simulink library "HexapodLocomotion_Library"  (R2023a)
settings: Solver=VariableStepAuto  StartTime=0.0  StopTime=10.0  RelTol=1e-3
values from neighbouring files (symbols this model uses):
  AEP = 0.03    [simulation_setup.m]
  max_torque_alpha = globalTorque    (= 0.94)    [InitialisationScript.m]    (also in simulation_setup.m)
  max_torque_beta = globalTorque    (= 0.94)    [InitialisationScript.m]    (also in simulation_setup.m)
  max_torque_gamma = globalTorque    (= 0.94)    [InitialisationScript.m]    (also in simulation_setup.m)
  N = 16    [rl_setup.m]
  PEP = -0.03    [simulation_setup.m]
  pid_D = 1    [InitialisationScript.m]    (also in simulation_setup.m)
  pid_filter_N = 100    [InitialisationScript.m]    (also in simulation_setup.m = 1000)
  pid_I = 0.2    [InitialisationScript.m]    (also in simulation_setup.m = 0.1)
  pid_P = 3    [InitialisationScript.m]    (also in simulation_setup.m = 600)
  step_height = 0.06    [InitialisationScript.m]    (also in simulation_setup.m)
  step_length = 0.04    [InitialisationScript.m]    (also in simulation_setup.m)
undefined symbols (not defined in the file or in its folder): X, Y, Z
libraries: sm_lib x31, nesl_utility x13, $bdroot x5, slpidlib x3
(part 1 of 2)
settings Model: Creator=basti  LastModifiedBy=basti

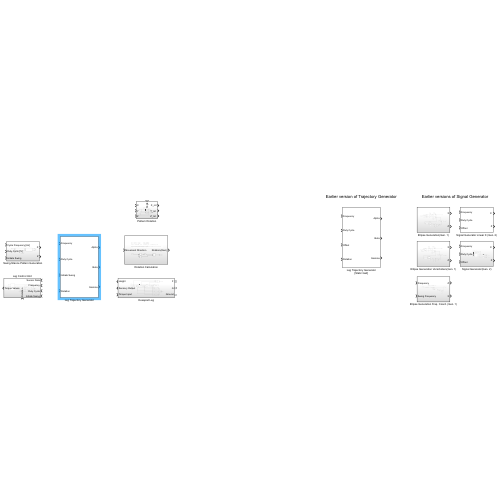
[thumbnail: Simulink's stored preview of the top-level diagram]
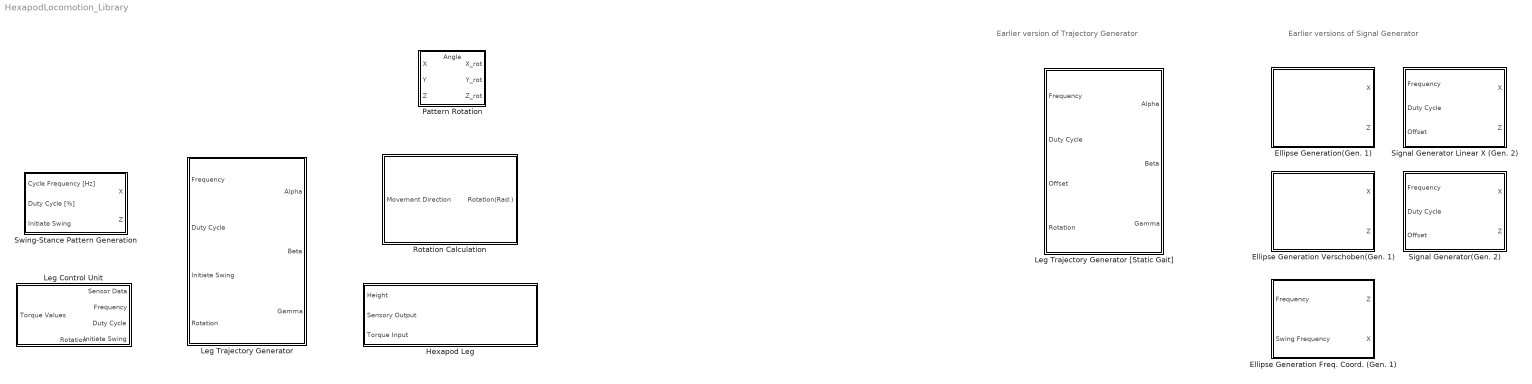
== system HexapodLocomotion_Library ==
  note: Earlier versions of Signal Generator
  note: Earlier version of Trajectory Generator
  Ellipse Generation Freq. Coord. (Gen. 1) : Subsystem
  Ellipse Generation Verschoben(Gen. 1) : Subsystem
  Ellipse Generation(Gen. 1) : Subsystem
  Hexapod Leg : Subsystem
      settings: PortSchema="{\"entries\":[{\"content\":{\"sides\":[{\"content\":{\"connectorIds\":[\"LConn1\",\"LConn2\",\"LConn3\"]},\"type\":\"ConnectorPlacement.EquallySpacedRectSide\",\"uuid\":\"f49879d6-ba76-4ec0-9cde-e27e7d64cb43\"},{\"content\":{\"connectorIds\":[\"In1\",\"Out1\",\"Out2\"],\"side\":\"RIGHT\"},\"type\":\"ConnectorPlacement.EquallySpacedRectSide\",\"uuid\":\"65b15dde-e5d7-47cb-8ac1-e9e029e05721\"},{\"content\":{\"side\":\"TOP\"},\"type\":\"ConnectorPlacement.EquallySpacedRectSide\",\"uuid\":\"11559e5b-a1be-4233-aeb2-21e170c4e963\"}]},\"type\":\"ConnectorPlacement.EquallySpacedConnector\",\"uuid\":\"c4377ad5-9946-4ac5-9145-d9e25f76b3b4\"}],\"packageUris\":[\"http://schema.mathworks.com/mf0/Connector/R2020b\"],\"version\":\"1.0\"}"
  Leg Control Unit : Subsystem
      settings: PortSchema="{\"entries\":[{\"content\":{\"sides\":[{\"content\":{\"connectorIds\":[\"In1\",\"In2\",\"In3\",\"In4\"]},\"type\":\"ConnectorPlacement.EquallySpacedRectSide\",\"uuid\":\"61807659-790a-4fcc-8eea-bb1747959d2c\"},{\"content\":{\"connectorIds\":[\"Out1\"],\"side\":\"RIGHT\"},\"type\":\"ConnectorPlacement.EquallySpacedRectSide\",\"uuid\":\"beab48f8-df50-4720-a4fe-1084d91255e1\"},{\"content\":{\"side\":\"TOP\"},\"type\":\"ConnectorPlacement.EquallySpacedRectSide\",\"uuid\":\"df2f0e11-b286-4413-8948-937711258f59\"},{\"content\":{\"connectorIds\":[\"In5\"],\"side\":\"BOTTOM\"},\"type\":\"ConnectorPlacement.EquallySpacedRectSide\",\"uuid\":\"177fd513-fdd6-4ae0-8805-86acc5cb073f\"}]},\"type\":\"ConnectorPlacement.EquallySpacedConnector\",\"uuid\":\"735c34ff-c8fb-4d96-b4d8-f985913f524f\"}],\"packageUris\":[\"http://schema.mathworks.com/mf0/Connector/R2020b\"],\"version\":\"1.0\"}"
  Leg Trajectory Generator : Subsystem  mask{step_height=0, step_length=0, x_offset=0, y_offset=0, z_offset=0, angle_offsets=0}
      mask prompts: step_height "Step Length"; step_length "Step Height"; x_offset "x-Offset"; y_offset "y-Offset"; z_offset "z-Offset"; angle_offsets "Angle Offsets"
  Leg Trajectory Generator [Static Gait] : Subsystem  mask{step_height=0, step_length=0, x_offset=0, y_offset=0, z_offset=0, angle_offsets=0}
      mask prompts: step_height "Step Length"; step_length "Step Height"; x_offset "x-Offset"; y_offset "y-Offset"; z_offset "z-Offset"; angle_offsets "Angle Offsets"
  Pattern Rotation : Subsystem
      settings: PortSchema="{\"entries\":[{\"content\":{\"sides\":[{\"content\":{\"connectorIds\":[\"In1\",\"In2\",\"In3\"]},\"type\":\"ConnectorPlacement.EquallySpacedRectSide\",\"uuid\":\"84b9b2e7-3aec-4c44-82b0-943baf46ecad\"},{\"content\":{\"connectorIds\":[\"Out1\",\"Out2\",\"Out3\"],\"side\":\"RIGHT\"},\"type\":\"ConnectorPlacement.EquallySpacedRectSide\",\"uuid\":\"b6460351-c898-40bb-b6f7-4663874c85b4\"},{\"content\":{\"connectorIds\":[\"In4\"],\"side\":\"TOP\"},\"type\":\"ConnectorPlacement.EquallySpacedRectSide\",\"uuid\":\"52dfc046-6500-4cf8-9639-535088e7a0e1\"}]},\"type\":\"ConnectorPlacement.EquallySpacedConnector\",\"uuid\":\"f9a3b501-bdbb-45c4-9129-59c2d41cd802\"}],\"packageUris\":[\"http://schema.mathworks.com/mf0/Connector/R2020b\"],\"version\":\"1.0\"}"
  Rotation Calculation : Subsystem
  Signal Generator Linear X (Gen. 2) : Subsystem  mask{x_amplitude=0, z_amplitude=0}
      mask prompts: x_amplitude "x-Amplitude"; z_amplitude "z-Amplitude"
  Signal Generator(Gen. 2) : Subsystem
  Swing-Stance Pattern Generation : Subsystem

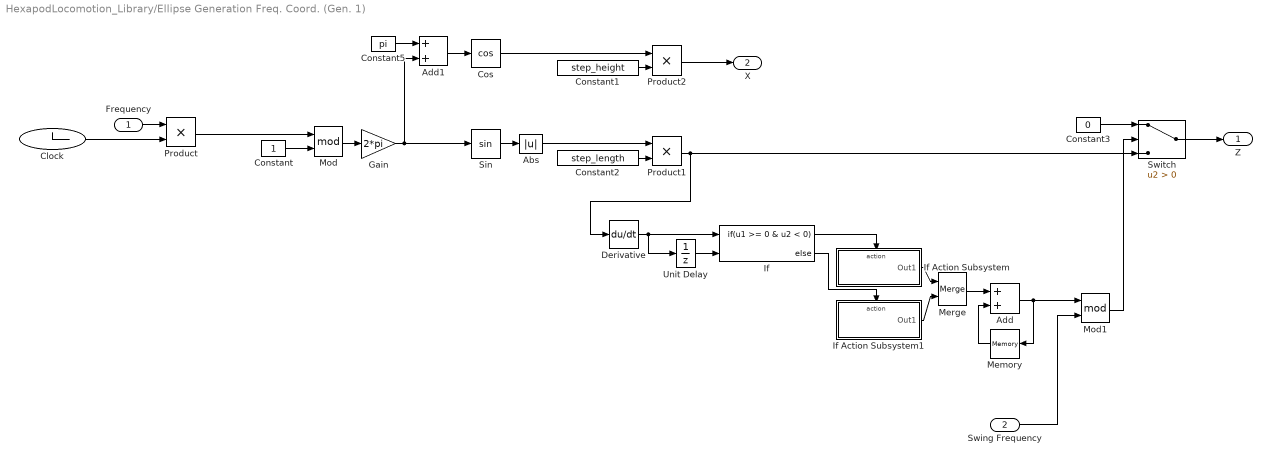
== system HexapodLocomotion_Library/Ellipse Generation Freq. Coord. (Gen. 1) ==
  Frequency : Inport
  Swing Frequency : Inport  Port=2
  Abs : Abs  SaturateOnIntegerOverflow=off
  Add : Sum
  Add1 : Sum
  Clock : Clock
  Constant : Constant
  Constant1 : Constant  Value=step_height
  Constant2 : Constant  Value=step_length
  Constant3 : Constant  Value=0
  Constant5 : Constant  Value=pi
  Cos : Trigonometry  Operator=cos
  Derivative : Derivative
  Gain : Gain  Gain=2*pi
  If : If  NumInputs=2  IfExpression=u1 >= 0 & u2 < 0
  If Action Subsystem : Subsystem  TreatAsAtomicUnit=on
  If Action Subsystem1 : Subsystem  TreatAsAtomicUnit=on
  Memory : Memory
  Merge : Merge
  Mod : Math  Operator=mod
  Mod1 : Math  Operator=mod
  Product : Product
  Product1 : Product
  Product2 : Product
  Sin : Trigonometry
  Switch : Switch  Criteria=u2 > Threshold  SaturateOnIntegerOverflow=off  InputSameDT=off
  Unit Delay : UnitDelay  SampleTime=-1  HasFrameUpgradeWarning=on
  Z : Outport
  X : Outport  Port=2
  wires:
  Clock/1 -> Product/2
  Frequency/1 -> Product/1
  Product/1 -> Mod/1
  Constant/1 -> Mod/2
  Mod/1 -> Gain/1
  Sin/1 -> Abs/1
  Constant2/1 -> Product1/2
  Cos/1 -> Product2/1
  Constant1/1 -> Product2/2
  Product1/1 -> Switch/3, Derivative/1
  Constant3/1 -> Switch/1
  Abs/1 -> Product1/1
  Derivative/1 -> Unit Delay/1, If/1
  Unit Delay/1 -> If/2
  If/2 -> If Action Subsystem1/Action
  If/1 -> If Action Subsystem/Action
  If Action Subsystem/1(Out1) -> Merge/1
  If Action Subsystem1/1(Out1) -> Merge/2
  Switch/1 -> Z/1
  Product2/1 -> X/1
  Merge/1 -> Add/1
  Memory/1 -> Add/2
  Add/1 -> Mod1/1, Memory/1
  Swing Frequency/1 -> Mod1/2
  Mod1/1 -> Switch/2
  Add1/1 -> Cos/1
  Constant5/1 -> Add1/1
  Gain/1 -> Add1/2, Sin/1

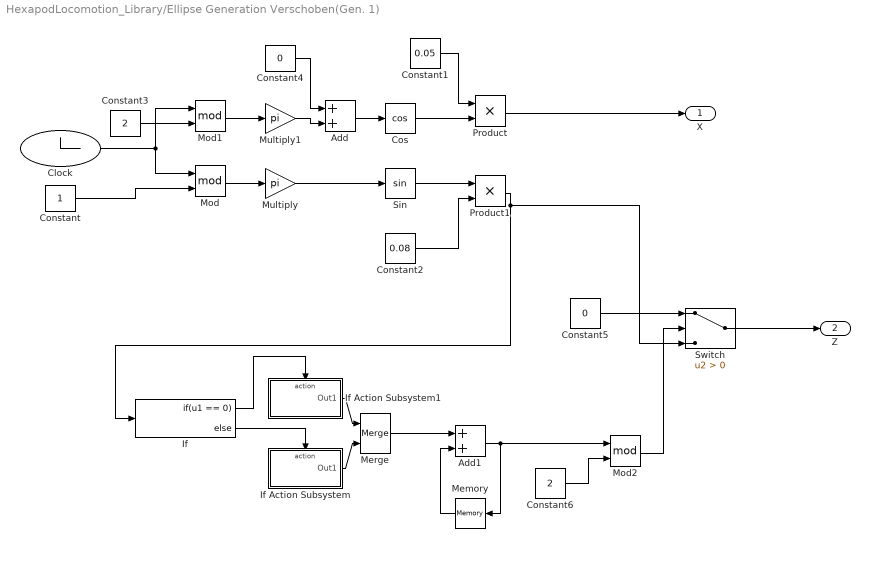
== system HexapodLocomotion_Library/Ellipse Generation Verschoben(Gen. 1) ==
  Add : Sum
  Add1 : Sum
  Clock : Clock
  Constant : Constant
  Constant1 : Constant  Value=0.05
  Constant2 : Constant  Value=0.08
  Constant3 : Constant  Value=2
  Constant4 : Constant  Value=0
  Constant5 : Constant  Value=0
  Constant6 : Constant  Value=2
  Cos : Trigonometry  Operator=cos
  If : If  IfExpression=u1 == 0
  If Action Subsystem : Subsystem  TreatAsAtomicUnit=on
  If Action Subsystem1 : Subsystem  TreatAsAtomicUnit=on
  Memory : Memory
  Merge : Merge
  Mod : Math  Operator=mod
  Mod1 : Math  Operator=mod
  Mod2 : Math  Operator=mod
  Multiply : Gain  Gain=pi
  Multiply1 : Gain  Gain=pi
  Product : Product
  Product1 : Product
  Sin : Trigonometry
  Switch : Switch  Criteria=u2 > Threshold  SaturateOnIntegerOverflow=off  InputSameDT=off
  X : Outport
  Z : Outport  Port=2
  wires:
  Clock/1 -> Mod1/1, Mod/1
  Constant/1 -> Mod/2
  Mod/1 -> Multiply/1
  Multiply/1 -> Sin/1
  Sin/1 -> Product1/1
  Cos/1 -> Product/2
  Constant1/1 -> Product/1
  Constant2/1 -> Product1/2
  Product1/1 -> Switch/3, If/1
  Product/1 -> X/1
  Mod1/1 -> Multiply1/1
  Constant3/1 -> Mod1/2
  Add/1 -> Cos/1
  Multiply1/1 -> Add/2
  Constant4/1 -> Add/1
  Add1/1 -> Mod2/1, Memory/1
  Memory/1 -> Add1/2
  If/2 -> If Action Subsystem/Action
  If/1 -> If Action Subsystem1/Action
  If Action Subsystem/1(Out1) -> Merge/2
  If Action Subsystem1/1(Out1) -> Merge/1
  Merge/1 -> Add1/1
  Switch/1 -> Z/1
  Constant5/1 -> Switch/1
  Constant6/1 -> Mod2/2
  Mod2/1 -> Switch/2

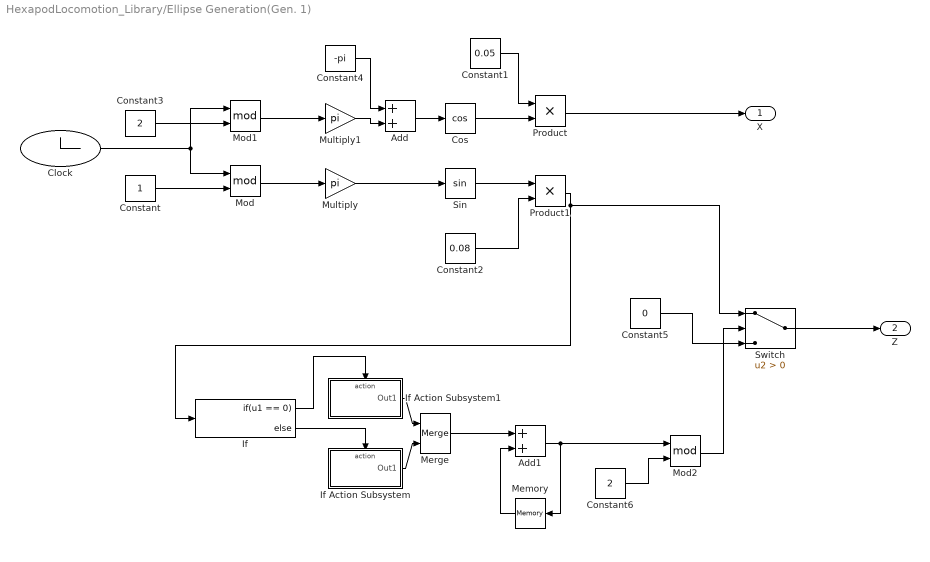
== system HexapodLocomotion_Library/Ellipse Generation(Gen. 1) ==
  Add : Sum
  Add1 : Sum
  Clock : Clock
  Constant : Constant
  Constant1 : Constant  Value=0.05
  Constant2 : Constant  Value=0.08
  Constant3 : Constant  Value=2
  Constant4 : Constant  Value=-pi
  Constant5 : Constant  Value=0
  Constant6 : Constant  Value=2
  Cos : Trigonometry  Operator=cos
  If : If  IfExpression=u1 == 0
  If Action Subsystem : Subsystem  TreatAsAtomicUnit=on
  If Action Subsystem1 : Subsystem  TreatAsAtomicUnit=on
  Memory : Memory
  Merge : Merge
  Mod : Math  Operator=mod
  Mod1 : Math  Operator=mod
  Mod2 : Math  Operator=mod
  Multiply : Gain  Gain=pi
  Multiply1 : Gain  Gain=pi
  Product : Product
  Product1 : Product
  Sin : Trigonometry
  Switch : Switch  Criteria=u2 > Threshold  SaturateOnIntegerOverflow=off  InputSameDT=off
  X : Outport
  Z : Outport  Port=2
  wires:
  Clock/1 -> Mod1/1, Mod/1
  Constant/1 -> Mod/2
  Mod/1 -> Multiply/1
  Multiply/1 -> Sin/1
  Sin/1 -> Product1/1
  Cos/1 -> Product/2
  Constant1/1 -> Product/1
  Constant2/1 -> Product1/2
  Product1/1 -> Switch/1, If/1
  Product/1 -> X/1
  Mod1/1 -> Multiply1/1
  Constant3/1 -> Mod1/2
  Add/1 -> Cos/1
  Multiply1/1 -> Add/2
  Constant4/1 -> Add/1
  Add1/1 -> Mod2/1, Memory/1
  Memory/1 -> Add1/2
  If/2 -> If Action Subsystem/Action
  If/1 -> If Action Subsystem1/Action
  If Action Subsystem/1(Out1) -> Merge/2
  If Action Subsystem1/1(Out1) -> Merge/1
  Merge/1 -> Add1/1
  Switch/1 -> Z/1
  Constant5/1 -> Switch/3
  Constant6/1 -> Mod2/2
  Mod2/1 -> Switch/2

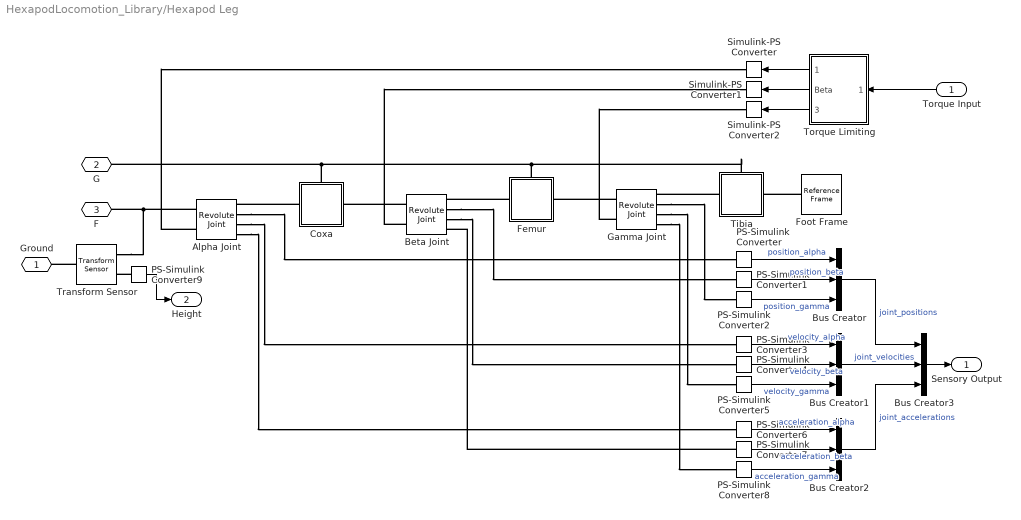
== system HexapodLocomotion_Library/Hexapod Leg ==
  Torque Input : Inport
  Alpha Joint : sm_lib/Joints/Revolute Joint  JointMode=Normal  SenseConstraintForce=off  SenseConstraintForceX=off  SenseConstraintForceY=off  SenseConstraintForceZ=off  SenseConstraintTorque=off  SenseConstraintTorqueX=off  SenseConstraintTorqueY=off  SenseConstraintTorqueZ=off  SenseTotalForce=off  SenseTotalForceX=off  SenseTotalForceY=off  SenseTotalForceZ=off  SenseTotalTorque=off  SenseTotalTorqueX=off  SenseTotalTorqueY=off  SenseTotalTorqueZ=off  CompositeWrenchDir=FollowerOnBase  CompositeWrenchFrame=BaseFrame  EquilibriumPosition=0  EquilibriumPositionUnits=deg  SpringStiffness=0  SpringStiffnessUnits=N*m/deg  DampingCoefficient=joint_damping_coefficient  DampingCoefficientUnits=kg*m^2/(rad*s)  TorqueActuationMode=InputTorque  MotionActuationMode=ComputedMotion  SensePosition=on  SenseVelocity=on  SenseAcceleration=on  SenseTorqueForce=off  SenseLowerLimitTorqueForce=off  SenseUpperLimitTorqueForce=off  LowerLimitSpecify=on  LowerLimitBound=-0.9599310885968813  LowerLimitBoundUnits=rad  LowerLimitStiffness=1e4  LowerLimitStiffnessUnits=N*m/deg  LowerLimitDamping=10  LowerLimitDampingUnits=N*m/(deg/s)  LowerLimitTransitionRegionWidth=global_transition_region  LowerLimitTransitionRegionWidthUnits=deg  UpperLimitSpecify=on  UpperLimitBound=0.9599310885968813  UpperLimitBoundUnits=rad  UpperLimitStiffness=1e4  UpperLimitStiffnessUnits=N*m/deg  UpperLimitDamping=10  UpperLimitDampingUnits=N*m/(deg/s)  UpperLimitTransitionRegionWidth=global_transition_region  UpperLimitTransitionRegionWidthUnits=deg  PositionTargetSpecify=on  PositionTargetPriority=High  PositionTargetValue=0  PositionTargetValueUnits=rad  VelocityTargetSpecify=off  VelocityTargetPriority=High  VelocityTargetValue=0  VelocityTargetValueUnits=deg/s
  Beta Joint : sm_lib/Joints/Revolute Joint  JointMode=Normal  SenseConstraintForce=off  SenseConstraintForceX=off  SenseConstraintForceY=off  SenseConstraintForceZ=off  SenseConstraintTorque=off  SenseConstraintTorqueX=off  SenseConstraintTorqueY=off  SenseConstraintTorqueZ=off  SenseTotalForce=off  SenseTotalForceX=off  SenseTotalForceY=off  SenseTotalForceZ=off  SenseTotalTorque=off  SenseTotalTorqueX=off  SenseTotalTorqueY=off  SenseTotalTorqueZ=off  CompositeWrenchDir=FollowerOnBase  CompositeWrenchFrame=BaseFrame  EquilibriumPosition=0  EquilibriumPositionUnits=deg  SpringStiffness=0  SpringStiffnessUnits=N*m/deg  DampingCoefficient=joint_damping_coefficient  DampingCoefficientUnits=kg*m^2/(rad*s)  TorqueActuationMode=InputTorque  MotionActuationMode=ComputedMotion  SensePosition=on  SenseVelocity=on  SenseAcceleration=on  SenseTorqueForce=off  SenseLowerLimitTorqueForce=off  SenseUpperLimitTorqueForce=off  LowerLimitSpecify=on  LowerLimitBound=-1.710422666954443  LowerLimitBoundUnits=rad  LowerLimitStiffness=1e4  LowerLimitStiffnessUnits=N*m/deg  LowerLimitDamping=10  LowerLimitDampingUnits=N*m/(deg/s)  LowerLimitTransitionRegionWidth=global_transition_region  LowerLimitTransitionRegionWidthUnits=deg  UpperLimitSpecify=on  UpperLimitBound=1.570796326794897  UpperLimitBoundUnits=rad  UpperLimitStiffness=1e4  UpperLimitStiffnessUnits=N*m/deg  UpperLimitDamping=10  UpperLimitDampingUnits=N*m/(deg/s)  UpperLimitTransitionRegionWidth=global_transition_region  UpperLimitTransitionRegionWidthUnits=deg  PositionTargetSpecify=on  PositionTargetPriority=High  PositionTargetValue=0  PositionTargetValueUnits=rad  VelocityTargetSpecify=off  VelocityTargetPriority=High  VelocityTargetValue=0  VelocityTargetValueUnits=deg/s
  Bus Creator{,1..3} (4 alike) : BusCreator  Inputs=3
  Coxa : Subsystem
      settings: PortSchema="{\"entries\":[{\"content\":{\"sides\":[{\"content\":{\"connectorIds\":[\"LConn1\"]},\"type\":\"ConnectorPlacement.EquallySpacedRectSide\",\"uuid\":\"688cd827-d904-4215-b5db-99d415378c46\"},{\"content\":{\"connectorIds\":[\"RConn1\"],\"side\":\"RIGHT\"},\"type\":\"ConnectorPlacement.EquallySpacedRectSide\",\"uuid\":\"69dd1601-faac-4bb0-843f-c649d8ea5326\"},{\"content\":{\"connectorIds\":[\"LConn2\"],\"side\":\"TOP\"},\"type\":\"ConnectorPlacement.EquallySpacedRectSide\",\"uuid\":\"f0d3334d-4e2f-4a21-b3dd-fad9d1fa7157\"}]},\"type\":\"ConnectorPlacement.EquallySpacedConnector\",\"uuid\":\"68f70a25-3d71-4639-b68a-a87509eaa3ad\"}],\"packageUris\":[\"http://schema.mathworks.com/mf0/Connector/R2020b\"],\"version\":\"1.0\"}"
  Femur : Subsystem
      settings: PortSchema="{\"entries\":[{\"content\":{\"sides\":[{\"content\":{\"connectorIds\":[\"LConn1\"]},\"type\":\"ConnectorPlacement.EquallySpacedRectSide\",\"uuid\":\"688cd827-d904-4215-b5db-99d415378c46\"},{\"content\":{\"connectorIds\":[\"RConn1\"],\"side\":\"RIGHT\"},\"type\":\"ConnectorPlacement.EquallySpacedRectSide\",\"uuid\":\"69dd1601-faac-4bb0-843f-c649d8ea5326\"},{\"content\":{\"connectorIds\":[\"LConn2\"],\"side\":\"TOP\"},\"type\":\"ConnectorPlacement.EquallySpacedRectSide\",\"uuid\":\"f0d3334d-4e2f-4a21-b3dd-fad9d1fa7157\"}]},\"type\":\"ConnectorPlacement.EquallySpacedConnector\",\"uuid\":\"68f70a25-3d71-4639-b68a-a87509eaa3ad\"}],\"packageUris\":[\"http://schema.mathworks.com/mf0/Connector/R2020b\"],\"version\":\"1.0\"}"
  Foot Frame : sm_lib/Frames and Transforms/Reference Frame
  Gamma Joint : sm_lib/Joints/Revolute Joint  JointMode=Normal  SenseConstraintForce=off  SenseConstraintForceX=off  SenseConstraintForceY=off  SenseConstraintForceZ=off  SenseConstraintTorque=off  SenseConstraintTorqueX=off  SenseConstraintTorqueY=off  SenseConstraintTorqueZ=off  SenseTotalForce=off  SenseTotalForceX=off  SenseTotalForceY=off  SenseTotalForceZ=off  SenseTotalTorque=off  SenseTotalTorqueX=off  SenseTotalTorqueY=off  SenseTotalTorqueZ=off  CompositeWrenchDir=FollowerOnBase  CompositeWrenchFrame=BaseFrame  EquilibriumPosition=0  EquilibriumPositionUnits=deg  SpringStiffness=0  SpringStiffnessUnits=N*m/deg  DampingCoefficient=joint_damping_coefficient  DampingCoefficientUnits=kg*m^2/(rad*s)  TorqueActuationMode=InputTorque  MotionActuationMode=ComputedMotion  SensePosition=on  SenseVelocity=on  SenseAcceleration=on  SenseTorqueForce=off  SenseLowerLimitTorqueForce=off  SenseUpperLimitTorqueForce=off  LowerLimitSpecify=on  LowerLimitBound=-0.7853981633974483  LowerLimitBoundUnits=rad  LowerLimitStiffness=1e4  LowerLimitStiffnessUnits=N*m/deg  LowerLimitDamping=10  LowerLimitDampingUnits=N*m/(deg/s)  LowerLimitTransitionRegionWidth=global_transition_region  LowerLimitTransitionRegionWidthUnits=deg  UpperLimitSpecify=on  UpperLimitBound=2.181661564992912  UpperLimitBoundUnits=rad  UpperLimitStiffness=1e4  UpperLimitStiffnessUnits=N*m/deg  UpperLimitDamping=10  UpperLimitDampingUnits=N*m/(deg/s)  UpperLimitTransitionRegionWidth=global_transition_region  UpperLimitTransitionRegionWidthUnits=deg  PositionTargetSpecify=on  PositionTargetPriority=High  PositionTargetValue=0  PositionTargetValueUnits=rad  VelocityTargetSpecify=off  VelocityTargetPriority=High  VelocityTargetValue=0  VelocityTargetValueUnits=deg/s
  PS-Simulink Converter{,1..9} (10 alike) : nesl_utility/PS-Simulink Converter  PhysicalDomain=network_engine_domain  SubClassName=ps_output  LeftPortType=input  RightPortType=output  PseudoPeriodic=off  Frequencies=[]  VectorFormat=inherit  Unit=inherit  AffineConversion=off
  Simulink-PS Converter : nesl_utility/Simulink-PS Converter  PhysicalDomain=network_engine_domain  SubClassName=ps_input  LeftPortType=input  RightPortType=output  PseudoPeriodic=off  Frequencies=[]  NoiseDistribution=none  NoiseParameters=[]  Unit=1  AffineConversion=off  FilteringAndDerivatives=provide  SimscapeFilterOrder=1  InputFilterTimeConstant=0.001  UdotUserProvided=0
  Simulink-PS Converter1 : nesl_utility/Simulink-PS Converter  PhysicalDomain=network_engine_domain  SubClassName=ps_input  LeftPortType=input  RightPortType=output  PseudoPeriodic=off  Frequencies=[]  NoiseDistribution=none  NoiseParameters=[]  Unit=1  AffineConversion=off  FilteringAndDerivatives=provide  SimscapeFilterOrder=1  InputFilterTimeConstant=0.001  UdotUserProvided=0
  Simulink-PS Converter2 : nesl_utility/Simulink-PS Converter  PhysicalDomain=network_engine_domain  SubClassName=ps_input  LeftPortType=input  RightPortType=output  PseudoPeriodic=off  Frequencies=[]  NoiseDistribution=none  NoiseParameters=[]  Unit=1  AffineConversion=off  FilteringAndDerivatives=provide  SimscapeFilterOrder=1  InputFilterTimeConstant=0.001  UdotUserProvided=0
  Tibia : Subsystem
      settings: PortSchema="{\"entries\":[{\"content\":{\"sides\":[{\"content\":{\"connectorIds\":[\"LConn1\"]},\"type\":\"ConnectorPlacement.EquallySpacedRectSide\",\"uuid\":\"99a4fa88-2354-49bd-896b-e43e2625a35e\"},{\"content\":{\"connectorIds\":[\"RConn1\"],\"side\":\"RIGHT\"},\"type\":\"ConnectorPlacement.EquallySpacedRectSide\",\"uuid\":\"27b73151-d7dc-445f-a6d8-c3ae4140e18d\"},{\"content\":{\"connectorIds\":[\"LConn2\"],\"side\":\"TOP\"},\"type\":\"ConnectorPlacement.EquallySpacedRectSide\",\"uuid\":\"5ff52d7d-b215-4137-a6c5-45615f920964\"}]},\"type\":\"ConnectorPlacement.EquallySpacedConnector\",\"uuid\":\"86768a5d-0bed-4b52-bc94-3bd267854b00\"}],\"packageUris\":[\"http://schema.mathworks.com/mf0/Connector/R2020b\"],\"version\":\"1.0\"}"
  Torque Limiting : Subsystem
  Transform Sensor : sm_lib/Frames and Transforms/Transform Sensor  MeasurementFrame=World  RotationSequence=XYX  SenseAngle=off  SenseAxis=off  SenseQ=off  SenseR=off  SenseRotationSequence=off  SenseOmegaX=off  SenseOmegaY=off  SenseOmegaZ=off  SenseQDot=off  SenseRDot=off  SenseRotationSequenceDot=off  SenseAlphaX=off  SenseAlphaY=off  SenseAlphaZ=off  SenseQDDot=off  SenseRDDot=off  SenseX=off  SenseY=off  SenseZ=on  SenseRad=off  SenseAzim=off  SenseDist=off  SenseInc=off  SenseXDot=off  SenseYDot=off  SenseZDot=off  SenseRadDot=off  SenseAzimDot=off  SenseDistDot=off  SenseIncDot=off  SenseXDDot=off  SenseYDDot=off  SenseZDDot=off  SenseRadDDot=off  SenseAzimDDot=off  SenseDistDDot=off  SenseIncDDot=off
  Ground : PMIOPort  Side=Left
  G : PMIOPort  Port=2  Side=Left
  F : PMIOPort  Port=3  Side=Left
  Sensory Output : Outport
  Height : Outport  Port=2
  wires:
  Torque Input/1 -> Torque Limiting/1(Input)
  Torque Limiting/1(Alpha) -> Simulink-PS Converter/1
  Torque Limiting/2(Beta) -> Simulink-PS Converter1/1
  Torque Limiting/3(Gamma) -> Simulink-PS Converter2/1
  PS-Simulink Converter/1 -> Bus Creator/1  "position_alpha"
  PS-Simulink Converter1/1 -> Bus Creator/2  "position_beta"
  PS-Simulink Converter2/1 -> Bus Creator/3  "position_gamma"
  PS-Simulink Converter3/1 -> Bus Creator1/1  "velocity_alpha"
  PS-Simulink Converter4/1 -> Bus Creator1/2  "velocity_beta"
  PS-Simulink Converter5/1 -> Bus Creator1/3  "velocity_gamma"
  PS-Simulink Converter6/1 -> Bus Creator2/1  "acceleration_alpha"
  PS-Simulink Converter7/1 -> Bus Creator2/2  "acceleration_beta"
  PS-Simulink Converter8/1 -> Bus Creator2/3  "acceleration_gamma"
  Bus Creator1/1 -> Bus Creator3/2  "joint_velocities"
  Bus Creator3/1 -> Sensory Output/1
  Bus Creator/1 -> Bus Creator3/1  "joint_positions"
  Bus Creator2/1 -> Bus Creator3/3  "joint_accelerations"
  PS-Simulink Converter9/1 -> Height/1
  connections:
  Beta Joint/LConn1 -- Coxa/RConn1
  Tibia/LConn1 -- Gamma Joint/RConn1
  Alpha Joint/LConn1 -- Transform Sensor/RConn1 -- F/RConn1
  Coxa/LConn1 -- Alpha Joint/RConn1
  Gamma Joint/LConn1 -- Femur/RConn1
  Femur/LConn1 -- Beta Joint/RConn1
  Gamma Joint/RConn2 -- PS-Simulink Converter2/LConn1
  Beta Joint/RConn2 -- PS-Simulink Converter1/LConn1
  Alpha Joint/RConn2 -- PS-Simulink Converter/LConn1
  Gamma Joint/LConn2 -- Simulink-PS Converter2/RConn1
  Beta Joint/LConn2 -- Simulink-PS Converter1/RConn1
  Alpha Joint/LConn2 -- Simulink-PS Converter/RConn1
  Coxa/LConn2 -- Tibia/LConn2 -- Femur/LConn2 -- G/RConn1
  Alpha Joint/RConn3 -- PS-Simulink Converter3/LConn1
  Beta Joint/RConn3 -- PS-Simulink Converter4/LConn1
  Gamma Joint/RConn3 -- PS-Simulink Converter5/LConn1
  Alpha Joint/RConn4 -- PS-Simulink Converter6/LConn1
  PS-Simulink Converter7/LConn1 -- Beta Joint/RConn4
  Gamma Joint/RConn4 -- PS-Simulink Converter8/LConn1
  Foot Frame/RConn1 -- Tibia/RConn1
  Transform Sensor/LConn1 -- Ground/RConn1
  PS-Simulink Converter9/LConn1 -- Transform Sensor/RConn2

== system HexapodLocomotion_Library/Leg Control Unit ==
  Sensor Data : Inport
  Frequency : Inport  Port=2
  Duty Cycle : Inport  Port=3
  Initiate Swing : Inport  Port=4
  Rotation : Inport  Port=5
  Bus Creator1 : BusCreator  Inputs=3
  Bus Selector1 : BusSelector  OutputSignals=joint_positions.position_alpha,joint_positions.position_beta,joint_positions.position_gamma
  Leg Trajectory Generator : $bdroot/Leg Trajectory Generator  step_height=0  step_length=0  x_offset=0  y_offset=0  z_offset=0  angle_offsets=0
  PID Controller1 : slpidlib/PID Controller  Controller=PID  Form=Parallel  TimeDomain=Continuous-time  UseExternalTs=off  SampleTime=-1  IntegratorMethod=Forward Euler  FilterMethod=Forward Euler  ControllerParametersSource=internal  P=pid_P  I=pid_I  UseKiTs=off  D=pid_D  N=pid_filter_N  UseFilter=on  TunerSelectOption=Transfer Function Based (PID Tuner App)  InitialConditionSource=internal  InitialConditionForIntegrator=0  InitialConditionForFilter=0  DifferentiatorICPrevScaledInput=0  ExternalReset=none  TrackingMode=off  Kt=1  LimitOutput=off  SatLimitsSource=internal  UpperSaturationLimit=inf  LowerSaturationLimit=-inf  LinearizeAsGain=on  AntiWindupMode=none  Kb=1  LimitIntegrator=off  UpperIntegratorSaturationLimit=inf  LowerIntegratorSaturationLimit=-inf  POutMin=[]  POutMax=[]  IOutMin=[]  IOutMax=[]  DOutMin=[]  DOutMax=[]  NOutMin=[]  NOutMax=[]  SumOutMin=[]  SumOutMax=[]  SaturationOutMin=[]  SaturationOutMax=[]  PParamMin=[]  PParamMax=[]  IParamMin=[]  IParamMax=[]  DParamMin=[]  DParamMax=[]  NParamMin=[]  NParamMax=[]  KbParamMin=[]  KbParamMax=[]  KtParamMin=[]  KtParamMax=[]  KbOutMin=[]  KbOutMax=[]  KtOutMin=[]  KtOutMax=[]  IntegratorOutMin=[]  IntegratorOutMax=[]  FilterOutMin=[]  FilterOutMax=[]  SumI1OutMin=[]  SumI1OutMax=[]  SumI2OutMin=[]  SumI2OutMax=[]  SumI3OutMin=[]  SumI3OutMax=[]  SumI4OutMin=[]  SumI4OutMax=[]  SumDOutMin=[]  SumDOutMax=[]  DifferentiatorOutMin=[]  DifferentiatorOutMax=[]  FilterDiffOutCoefMin=[]  FilterDiffOutCoefMax=[]  ReciprocalOutMin=[]  ReciprocalOutMax=[]  SumDenOutMin=[]  SumDenOutMax=[]  SumNumOutMin=[]  SumNumOutMax=[]  DivideOutMin=[]  DivideOutMax=[]  UdiffTsProdOutMin=[]  UdiffTsProdOutMax=[]  NTsProdOutMin=[]  NTsProdOutMax=[]  UintegralTsProdOutMin=[]  UintegralTsProdOutMax=[]  UngainTsProdOutMin=[]  UngainTsProdOutMax=[]  ClampingZeroOutDataTypeStr=Inherit: Inherit via back propagation  ClampingZeroOutMin=[]  ClampingZeroOutMax=[]  FilterDenConstantOutDataTypeStr=Inherit: Inherit via back propagation  FilterDenConstantOutMin=[]  FilterDenConstantOutMax=[]  PCopyOutDataTypeStr=Inherit: Inherit via back propagation  PCopyOutMin=[]  PCopyOutMax=[]  NCopyOutDataTypeStr=Inherit: Inherit via back propagation  NCopyOutMin=[]  NCopyOutMax=[]  IntegratorContinuousStateAttributes=''  IntegratorStateMustResolveToSignalObject=off  IntegratorRTWStateStorageClass=Auto  FilterContinuousStateAttributes=''  FilterStateMustResolveToSignalObject=off  FilterRTWStateStorageClass=Auto  ParallelPVariant=InternalParameters  IdealPVariant=Disabled  IVariant=InternalParameters  DVariant=InternalParameters  IntegratorVariant=Continuous  SatVariant=Disabled  AWVariant=Passthrough  PCopyVariant=Disabled  TRVariant=Disabled  FdbkBlocksVariant=Forward  IdealPFdbkVariant=Disabled  SatFdbkVariant=Disabled  DerivativeFilterVariant=ContFilter  NVariant=InternalParameters  NCopyVariant=Disabled  FilterICVariant=InternalICsFilter  IntegratorICVariant=InternalICs  ExternalResetVariant=Disabled  TRSumVariant=Passthrough  SumFdbkVariant=Disabled  SumVariant=Sum_PID  TsampFilterVariant=InternalTs  TsampNgainVariant=Passthrough  TsampIntegralVariant=Disabled_SignalSpec  ExternalSaturationOutDataTypeStr=Inherit: Same as second input
  PID Controller2 : slpidlib/PID Controller  Controller=PID  Form=Parallel  TimeDomain=Continuous-time  UseExternalTs=off  SampleTime=-1  IntegratorMethod=Forward Euler  FilterMethod=Forward Euler  ControllerParametersSource=internal  P=pid_P  I=pid_I  UseKiTs=off  D=pid_D  N=pid_filter_N  UseFilter=on  TunerSelectOption=Transfer Function Based (PID Tuner App)  InitialConditionSource=internal  InitialConditionForIntegrator=0  InitialConditionForFilter=0  DifferentiatorICPrevScaledInput=0  ExternalReset=none  TrackingMode=off  Kt=1  LimitOutput=off  SatLimitsSource=internal  UpperSaturationLimit=inf  LowerSaturationLimit=-inf  LinearizeAsGain=on  AntiWindupMode=none  Kb=1  LimitIntegrator=off  UpperIntegratorSaturationLimit=inf  LowerIntegratorSaturationLimit=-inf  POutMin=[]  POutMax=[]  IOutMin=[]  IOutMax=[]  DOutMin=[]  DOutMax=[]  NOutMin=[]  NOutMax=[]  SumOutMin=[]  SumOutMax=[]  SaturationOutMin=[]  SaturationOutMax=[]  PParamMin=[]  PParamMax=[]  IParamMin=[]  IParamMax=[]  DParamMin=[]  DParamMax=[]  NParamMin=[]  NParamMax=[]  KbParamMin=[]  KbParamMax=[]  KtParamMin=[]  KtParamMax=[]  KbOutMin=[]  KbOutMax=[]  KtOutMin=[]  KtOutMax=[]  IntegratorOutMin=[]  IntegratorOutMax=[]  FilterOutMin=[]  FilterOutMax=[]  SumI1OutMin=[]  SumI1OutMax=[]  SumI2OutMin=[]  SumI2OutMax=[]  SumI3OutMin=[]  SumI3OutMax=[]  SumI4OutMin=[]  SumI4OutMax=[]  SumDOutMin=[]  SumDOutMax=[]  DifferentiatorOutMin=[]  DifferentiatorOutMax=[]  FilterDiffOutCoefMin=[]  FilterDiffOutCoefMax=[]  ReciprocalOutMin=[]  ReciprocalOutMax=[]  SumDenOutMin=[]  SumDenOutMax=[]  SumNumOutMin=[]  SumNumOutMax=[]  DivideOutMin=[]  DivideOutMax=[]  UdiffTsProdOutMin=[]  UdiffTsProdOutMax=[]  NTsProdOutMin=[]  NTsProdOutMax=[]  UintegralTsProdOutMin=[]  UintegralTsProdOutMax=[]  UngainTsProdOutMin=[]  UngainTsProdOutMax=[]  ClampingZeroOutDataTypeStr=Inherit: Inherit via back propagation  ClampingZeroOutMin=[]  ClampingZeroOutMax=[]  FilterDenConstantOutDataTypeStr=Inherit: Inherit via back propagation  FilterDenConstantOutMin=[]  FilterDenConstantOutMax=[]  PCopyOutDataTypeStr=Inherit: Inherit via back propagation  PCopyOutMin=[]  PCopyOutMax=[]  NCopyOutDataTypeStr=Inherit: Inherit via back propagation  NCopyOutMin=[]  NCopyOutMax=[]  IntegratorContinuousStateAttributes=''  IntegratorStateMustResolveToSignalObject=off  IntegratorRTWStateStorageClass=Auto  FilterContinuousStateAttributes=''  FilterStateMustResolveToSignalObject=off  FilterRTWStateStorageClass=Auto  ParallelPVariant=InternalParameters  IdealPVariant=Disabled  IVariant=InternalParameters  DVariant=InternalParameters  IntegratorVariant=Continuous  SatVariant=Disabled  AWVariant=Passthrough  PCopyVariant=Disabled  TRVariant=Disabled  FdbkBlocksVariant=Forward  IdealPFdbkVariant=Disabled  SatFdbkVariant=Disabled  DerivativeFilterVariant=ContFilter  NVariant=InternalParameters  NCopyVariant=Disabled  FilterICVariant=InternalICsFilter  IntegratorICVariant=InternalICs  ExternalResetVariant=Disabled  TRSumVariant=Passthrough  SumFdbkVariant=Disabled  SumVariant=Sum_PID  TsampFilterVariant=InternalTs  TsampNgainVariant=Passthrough  TsampIntegralVariant=Disabled_SignalSpec  ExternalSaturationOutDataTypeStr=Inherit: Same as second input
  PID Controller3 : slpidlib/PID Controller  Controller=PID  Form=Parallel  TimeDomain=Continuous-time  UseExternalTs=off  SampleTime=-1  IntegratorMethod=Forward Euler  FilterMethod=Forward Euler  ControllerParametersSource=internal  P=pid_P  I=pid_I  UseKiTs=off  D=pid_D  N=pid_filter_N  UseFilter=on  TunerSelectOption=Transfer Function Based (PID Tuner App)  InitialConditionSource=internal  InitialConditionForIntegrator=0  InitialConditionForFilter=0  DifferentiatorICPrevScaledInput=0  ExternalReset=none  TrackingMode=off  Kt=1  LimitOutput=off  SatLimitsSource=internal  UpperSaturationLimit=inf  LowerSaturationLimit=-inf  LinearizeAsGain=on  AntiWindupMode=none  Kb=1  LimitIntegrator=off  UpperIntegratorSaturationLimit=inf  LowerIntegratorSaturationLimit=-inf  POutMin=[]  POutMax=[]  IOutMin=[]  IOutMax=[]  DOutMin=[]  DOutMax=[]  NOutMin=[]  NOutMax=[]  SumOutMin=[]  SumOutMax=[]  SaturationOutMin=[]  SaturationOutMax=[]  PParamMin=[]  PParamMax=[]  IParamMin=[]  IParamMax=[]  DParamMin=[]  DParamMax=[]  NParamMin=[]  NParamMax=[]  KbParamMin=[]  KbParamMax=[]  KtParamMin=[]  KtParamMax=[]  KbOutMin=[]  KbOutMax=[]  KtOutMin=[]  KtOutMax=[]  IntegratorOutMin=[]  IntegratorOutMax=[]  FilterOutMin=[]  FilterOutMax=[]  SumI1OutMin=[]  SumI1OutMax=[]  SumI2OutMin=[]  SumI2OutMax=[]  SumI3OutMin=[]  SumI3OutMax=[]  SumI4OutMin=[]  SumI4OutMax=[]  SumDOutMin=[]  SumDOutMax=[]  DifferentiatorOutMin=[]  DifferentiatorOutMax=[]  FilterDiffOutCoefMin=[]  FilterDiffOutCoefMax=[]  ReciprocalOutMin=[]  ReciprocalOutMax=[]  SumDenOutMin=[]  SumDenOutMax=[]  SumNumOutMin=[]  SumNumOutMax=[]  DivideOutMin=[]  DivideOutMax=[]  UdiffTsProdOutMin=[]  UdiffTsProdOutMax=[]  NTsProdOutMin=[]  NTsProdOutMax=[]  UintegralTsProdOutMin=[]  UintegralTsProdOutMax=[]  UngainTsProdOutMin=[]  UngainTsProdOutMax=[]  ClampingZeroOutDataTypeStr=Inherit: Inherit via back propagation  ClampingZeroOutMin=[]  ClampingZeroOutMax=[]  FilterDenConstantOutDataTypeStr=Inherit: Inherit via back propagation  FilterDenConstantOutMin=[]  FilterDenConstantOutMax=[]  PCopyOutDataTypeStr=Inherit: Inherit via back propagation  PCopyOutMin=[]  PCopyOutMax=[]  NCopyOutDataTypeStr=Inherit: Inherit via back propagation  NCopyOutMin=[]  NCopyOutMax=[]  IntegratorContinuousStateAttributes=''  IntegratorStateMustResolveToSignalObject=off  IntegratorRTWStateStorageClass=Auto  FilterContinuousStateAttributes=''  FilterStateMustResolveToSignalObject=off  FilterRTWStateStorageClass=Auto  ParallelPVariant=InternalParameters  IdealPVariant=Disabled  IVariant=InternalParameters  DVariant=InternalParameters  IntegratorVariant=Continuous  SatVariant=Disabled  AWVariant=Passthrough  PCopyVariant=Disabled  TRVariant=Disabled  FdbkBlocksVariant=Forward  IdealPFdbkVariant=Disabled  SatFdbkVariant=Disabled  DerivativeFilterVariant=ContFilter  NVariant=InternalParameters  NCopyVariant=Disabled  FilterICVariant=InternalICsFilter  IntegratorICVariant=InternalICs  ExternalResetVariant=Disabled  TRSumVariant=Passthrough  SumFdbkVariant=Disabled  SumVariant=Sum_PID  TsampFilterVariant=InternalTs  TsampNgainVariant=Passthrough  TsampIntegralVariant=Disabled_SignalSpec  ExternalSaturationOutDataTypeStr=Inherit: Same as second input
  Sum1 : Sum  Inputs=|+-
  Sum2 : Sum  Inputs=|+-
  Sum3 : Sum  Inputs=|+-
  Torque Values : Outport
  wires:
  Frequency/1 -> Leg Trajectory Generator/1
  Initiate Swing/1 -> Leg Trajectory Generator/3
  Duty Cycle/1 -> Leg Trajectory Generator/2
  PID Controller2/1 -> Bus Creator1/2  "torque_beta"
  Sensor Data/1 -> Bus Selector1/1
  Bus Creator1/1 -> Torque Values/1
  Leg Trajectory Generator/1 -> Sum1/1
  Leg Trajectory Generator/3 -> Sum3/1
  Leg Trajectory Generator/2 -> Sum2/1
  Bus Selector1/3 -> Sum3/2  "<position_gamma>"
  Bus Selector1/2 -> Sum2/2  "<position_beta>"
  Sum3/1 -> PID Controller3/1
  PID Controller3/1 -> Bus Creator1/3  "torque_gamma"
  PID Controller1/1 -> Bus Creator1/1  "torque_alpha"
  Bus Selector1/1 -> Sum1/2  "<position_alpha>"
  Sum2/1 -> PID Controller2/1
  Sum1/1 -> PID Controller1/1
  Rotation/1 -> Leg Trajectory Generator/4

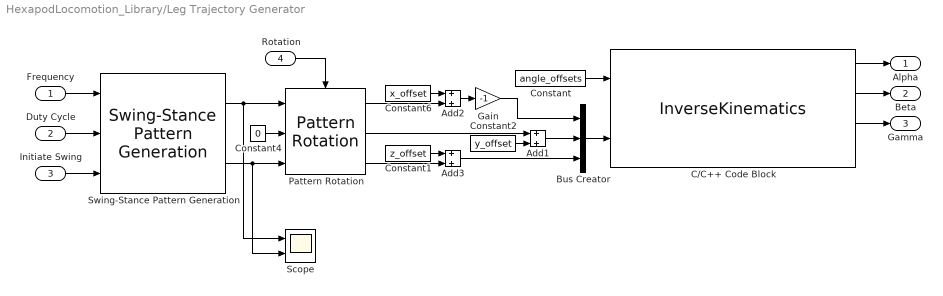
== system HexapodLocomotion_Library/Leg Trajectory Generator ==
  Frequency : Inport
  Duty Cycle : Inport  Port=2
  Initiate Swing : Inport  Port=3
  Rotation : Inport  Port=4
  Add1 : Sum
  Add2 : Sum
  Add3 : Sum
  Bus Creator : BusCreator  Inputs=3
  C/C++ Code Block : S-Function  FunctionName=InverseKinematics  SFunctionModules=InverseKinematics_wrapper.c  SFunctionDeploymentMode=off  EnableBusSupport=off  mask(S-Function Builder){}
      mask help: Simulink:masks:SFunctionBuilder_MD
      mask init:
      | val = [[.9  0.75 0.75 1 1 .9 .9 1]',[1 1 0.75 0.75 .9 .9 1 .9]'];try , sys = get_param(gcb,'SfunBuilderFcnName');if isempty(sys), sys = get_param(gcb,'FunctionName'); end,catch, sys = get_param(gcb,'FunctionName'); end
      settings: CopyFcn=set_param(gcbh,'LinkStatus','none')  OpenFcn=sfunctionwizard(gcbh)
      mask Display:
      | plot(val(:,1),val(:,2))
      | disp(sys)
      | port_label('input',1,'angle_offsets')
      | port_label('input',2,'coordinates')
      | port_label('output',1,'alpha')
      | port_label('output',2,'beta')
      | port_label('output',3,'gamma')
      | port_label('output',4,'debug')
  Constant : Constant  Value=angle_offsets
  Constant1 : Constant  Value=z_offset
  Constant2 : Constant  Value=y_offset
  Constant4 : Constant  Value=0
  Constant6 : Constant  Value=x_offset
  Gain : Gain  Gain=-1
  Pattern Rotation : $bdroot/Pattern Rotation  SystemSampleTime=-1  VariantActivationTime=update diagram  Latency=0  AutoFrameSizeCalculation=off
      settings: PortSchema="{\"entries\":[{\"content\":{\"sides\":[{\"content\":{\"connectorIds\":[\"In1\",\"In2\",\"In3\"]},\"type\":\"ConnectorPlacement.EquallySpacedRectSide\",\"uuid\":\"84b9b2e7-3aec-4c44-82b0-943baf46ecad\"},{\"content\":{\"connectorIds\":[\"Out1\",\"Out2\",\"Out3\"],\"side\":\"RIGHT\"},\"type\":\"ConnectorPlacement.EquallySpacedRectSide\",\"uuid\":\"b6460351-c898-40bb-b6f7-4663874c85b4\"},{\"content\":{\"connectorIds\":[\"In4\"],\"side\":\"TOP\"},\"type\":\"ConnectorPlacement.EquallySpacedRectSide\",\"uuid\":\"52dfc046-6500-4cf8-9639-535088e7a0e1\"}]},\"type\":\"ConnectorPlacement.EquallySpacedConnector\",\"uuid\":\"f9a3b501-bdbb-45c4-9129-59c2d41cd802\"}],\"packageUris\":[\"http://schema.mathworks.com/mf0/Connector/R2020b\"],\"version\":\"1.0\"}"
  Scope : Scope  NumInputPorts=2
  Swing-Stance Pattern Generation : $bdroot/Swing-Stance Pattern Generation  SystemSampleTime=-1  VariantActivationTime=update diagram  Latency=0  AutoFrameSizeCalculation=off
  Alpha : Outport
  Beta : Outport  Port=2
  Gamma : Outport  Port=3
  wires:
  C/C++ Code Block/3 -> Gamma/1
  C/C++ Code Block/2 -> Beta/1
  C/C++ Code Block/1 -> Alpha/1
  Bus Creator/1 -> C/C++ Code Block/2
  Constant/1 -> C/C++ Code Block/1
  Frequency/1 -> Swing-Stance Pattern Generation/1
  Duty Cycle/1 -> Swing-Stance Pattern Generation/2
  Gain/1 -> Bus Creator/1
  Add1/1 -> Bus Creator/2
  Add3/1 -> Bus Creator/3
  Add2/1 -> Gain/1
  Swing-Stance Pattern Generation/1 -> Pattern Rotation/1, Scope/1
  Pattern Rotation/1 -> Add2/2
  Swing-Stance Pattern Generation/2 -> Scope/2, Pattern Rotation/3
  Pattern Rotation/3 -> Add3/2
  Pattern Rotation/2 -> Add1/1
  Constant2/1 -> Add1/2
  Constant4/1 -> Pattern Rotation/2
  Constant6/1 -> Add2/1
  Constant1/1 -> Add3/1
  Initiate Swing/1 -> Swing-Stance Pattern Generation/3
  Rotation/1 -> Pattern Rotation/4

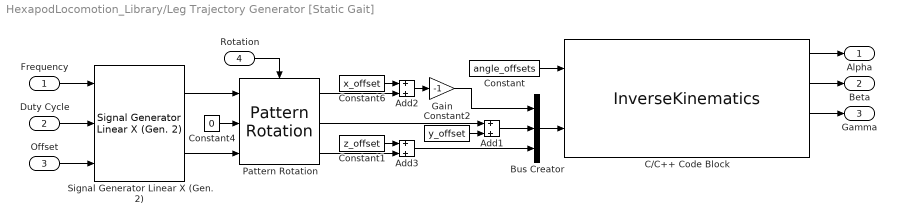
== system HexapodLocomotion_Library/Leg Trajectory Generator [Static Gait] ==
  Frequency : Inport
  Duty Cycle : Inport  Port=2
  Offset : Inport  Port=3
  Rotation : Inport  Port=4
  Add1 : Sum
  Add2 : Sum
  Add3 : Sum
  Bus Creator : BusCreator  Inputs=3
  C/C++ Code Block : S-Function  FunctionName=InverseKinematics  SFunctionModules=InverseKinematics_wrapper.c  SFunctionDeploymentMode=off  EnableBusSupport=off  mask(S-Function Builder){}
      mask help: Simulink:masks:SFunctionBuilder_MD
      mask init: same as HexapodLocomotion_Library/Leg Trajectory Generator/C/C++ Code Block
      settings: CopyFcn=set_param(gcbh,'LinkStatus','none')  OpenFcn=sfunctionwizard(gcbh)
      mask Display:
      | plot(val(:,1),val(:,2))
      | disp(sys)
      | port_label('input',1,'angle_offsets')
      | port_label('input',2,'coordinates')
      | port_label('output',1,'alpha')
      | port_label('output',2,'beta')
      | port_label('output',3,'gamma')
      | port_label('output',4,'debug')
  Constant : Constant  Value=angle_offsets
  Constant1 : Constant  Value=z_offset
  Constant2 : Constant  Value=y_offset
  Constant4 : Constant  Value=0
  Constant6 : Constant  Value=x_offset
  Gain : Gain  Gain=-1
  Pattern Rotation : $bdroot/Pattern Rotation  SystemSampleTime=-1  VariantActivationTime=update diagram  Latency=0  AutoFrameSizeCalculation=off
      settings: PortSchema="{\"entries\":[{\"content\":{\"sides\":[{\"content\":{\"connectorIds\":[\"In1\",\"In2\",\"In3\"]},\"type\":\"ConnectorPlacement.EquallySpacedRectSide\",\"uuid\":\"84b9b2e7-3aec-4c44-82b0-943baf46ecad\"},{\"content\":{\"connectorIds\":[\"Out1\",\"Out2\",\"Out3\"],\"side\":\"RIGHT\"},\"type\":\"ConnectorPlacement.EquallySpacedRectSide\",\"uuid\":\"b6460351-c898-40bb-b6f7-4663874c85b4\"},{\"content\":{\"connectorIds\":[\"In4\"],\"side\":\"TOP\"},\"type\":\"ConnectorPlacement.EquallySpacedRectSide\",\"uuid\":\"52dfc046-6500-4cf8-9639-535088e7a0e1\"}]},\"type\":\"ConnectorPlacement.EquallySpacedConnector\",\"uuid\":\"f9a3b501-bdbb-45c4-9129-59c2d41cd802\"}],\"packageUris\":[\"http://schema.mathworks.com/mf0/Connector/R2020b\"],\"version\":\"1.0\"}"
  Signal Generator Linear X (Gen. 2) : $bdroot/Signal Generator Linear X (Gen. 2)  x_amplitude=step_length/2  z_amplitude=step_height
  Alpha : Outport
  Beta : Outport  Port=2
  Gamma : Outport  Port=3
  wires:
  C/C++ Code Block/3 -> Gamma/1
  C/C++ Code Block/2 -> Beta/1
  C/C++ Code Block/1 -> Alpha/1
  Bus Creator/1 -> C/C++ Code Block/2
  Constant/1 -> C/C++ Code Block/1
  Frequency/1 -> Signal Generator Linear X (Gen. 2)/1
  Duty Cycle/1 -> Signal Generator Linear X (Gen. 2)/2
  Offset/1 -> Signal Generator Linear X (Gen. 2)/3
  Gain/1 -> Bus Creator/1
  Add1/1 -> Bus Creator/2
  Add3/1 -> Bus Creator/3
  Add2/1 -> Gain/1
  Rotation/1 -> Pattern Rotation/4
  Signal Generator Linear X (Gen. 2)/1 -> Pattern Rotation/1
  Pattern Rotation/1 -> Add2/2
  Signal Generator Linear X (Gen. 2)/2 -> Pattern Rotation/3
  Pattern Rotation/3 -> Add3/2
  Pattern Rotation/2 -> Add1/1
  Constant2/1 -> Add1/2
  Constant4/1 -> Pattern Rotation/2
  Constant6/1 -> Add2/1
  Constant1/1 -> Add3/1

== system HexapodLocomotion_Library/Pattern Rotation ==
  note: (2D-Rotation-Matrix):
      | x_new = x_old * cos(theta) - y_old*sin(theta)
      | y_new = x_old*sin(theta) + y_old*cos(theta)
  "X " : Inport
  Y : Inport  Port=2
  Z : Inport  Port=3
  Angle : Inport  Port=4
  Add : Sum
  Cos : Trigonometry  Operator=cos
  Cos1 : Trigonometry  Operator=cos
  Product{,1..2,4} (4 alike) : Product
  Sin : Trigonometry
  Sin1 : Trigonometry
  Subtract : Sum  Inputs=+-
  X_rot : Outport
  "Y_rot " : Outport  Port=2
  "Z_rot " : Outport  Port=3
  wires:
  Z/1 -> "Z_rot "/1
  Subtract/1 -> X_rot/1
  Add/1 -> "Y_rot "/1
  Product/1 -> Subtract/1
  Product1/1 -> Subtract/2
  Product2/1 -> Add/1
  Product4/1 -> Add/2
  Cos/1 -> Product/1
  "X "/1 -> Product2/2, Product/2
  Angle/1 -> Cos1/1, Sin1/1, Sin/1, Cos/1
  Y/1 -> Product1/2, Product4/2
  Sin/1 -> Product1/1
  Sin1/1 -> Product2/1
  Cos1/1 -> Product4/1

== system HexapodLocomotion_Library/Rotation Calculation ==
  note: dot = x1*x2 + y1*y2 # dot product
      | det = x1*y2 - y1*x2 # determinant
      | angle = atan2(det, dot) # atan2(y, x) or atan2(sin, cos)
      | https://math.stackexchange.com/questions/878785/how-to-find-an-angle-in-range0-360-between-2-vectors
  Movement Direction : Inport
  Atan2 : Trigonometry  Operator=atan2
  Gain : Gain  Gain=-1
  Selector2 : Selector  IndexMode=Zero-based  InputPortWidth=2  IndexOptions=Starting index (dialog)  Indices=0  OutputSizes=1  RuntimeRangeChecks=on
  Selector3 : Selector  IndexMode=Zero-based  InputPortWidth=2  IndexOptions=Starting index (dialog)  Indices=1  OutputSizes=1
  Rotation(Rad.) : Outport
  wires:
  Selector3/1 -> Atan2/2
  Atan2/1 -> Rotation(Rad.)/1
  Selector2/1 -> Gain/1
  Movement Direction/1 -> Selector3/1, Selector2/1
  Gain/1 -> Atan2/1

== system HexapodLocomotion_Library/Signal Generator Linear X (Gen. 2) ==
  note: (1/Hz) *duty_cycle = duty_cycle/Hz = swing_time
      |
      | 1/swing_time = 1 / (duty_cycle/Hz) = Hz/duty_cycle = Hz_for_swing
      | ----------------------------------------------------------------------------------------------------
      | (1/Hz)*(1-duty_cycle) = (1-duty_cycle)/Hz = stance_time
      |
      | 1/stance_time = 1 / ((1-duty_cycle)/Hz) = Hz / (1-duty_cycle) = Hz_for_stance
  Frequency : Inport
  Duty Cycle : Inport  Port=2
  Offset : Inport  Port=3
  Constant2 : Constant
  Divide : Product  Inputs=*/
  Divide1 : Product  Inputs=*/
  Gain : Gain  Gain=0.5
  Gain1 : Gain  Gain=0.5
  Stance Phase : Subsystem  TreatAsAtomicUnit=on
  Subsystem : Subsystem
  Subtract : Sum  Inputs=+-
  Swing Phase : Subsystem  TreatAsAtomicUnit=on
  Switch : Switch  Criteria=u2 > Threshold  SaturateOnIntegerOverflow=off  InputSameDT=off
  Switch1 : Switch  Criteria=u2 > Threshold  SaturateOnIntegerOverflow=off  InputSameDT=off
  "X " : Outport
  Z : Outport  Port=2
  wires:
  Swing Phase/1(X) -> Switch/1
  Swing Phase/2("Z ") -> Switch1/1
  Stance Phase/2("Z ") -> Switch1/3
  Stance Phase/1(X) -> Switch/3
  Divide1/1 -> Gain1/1
  Divide/1 -> Gain/1
  Duty Cycle/1 -> Divide/2, Subtract/2, Subsystem/2(Duty Cycle)
  Offset/1 -> Subsystem/3(Offset)
  Frequency/1 -> Divide/1, Divide1/1, Subsystem/1(Frequency)
  Subsystem/1(Swing Activation) -> Switch/2, Switch1/2, Swing Phase/Reset
  Subsystem/2(Stance Activation) -> Stance Phase/Reset
  Subtract/1 -> Divide1/2
  Constant2/1 -> Subtract/1
  Gain/1 -> Swing Phase/1(Frequency)
  Gain1/1 -> Stance Phase/1(Frequency)
  Switch1/1 -> Z/1
  Switch/1 -> "X "/1

== system HexapodLocomotion_Library/Signal Generator(Gen. 2) ==
  note: (1/Hz) *duty_cycle = duty_cycle/Hz = swing_time
      |
      | 1/swing_time = 1 / (duty_cycle/Hz) = Hz/duty_cycle = Hz_for_swing
      | ----------------------------------------------------------------------------------------------------
      | (1/Hz)*(1-duty_cycle) = (1-duty_cycle)/Hz = stance_time
      |
      | 1/stance_time = 1 / ((1-duty_cycle)/Hz) = Hz / (1-duty_cycle) = Hz_for_stance
  Frequency : Inport
  Duty Cycle : Inport  Port=2
  Offset : Inport  Port=3
  Constant2 : Constant
  Divide : Product  Inputs=*/
  Divide1 : Product  Inputs=*/
  Gain : Gain  Gain=0.5
  Gain1 : Gain  Gain=0.5
  Stance Phase : Subsystem  TreatAsAtomicUnit=on
  Subsystem : Subsystem
  Subtract : Sum  Inputs=+-
  Swing Phase : Subsystem  TreatAsAtomicUnit=on
  Switch : Switch  Criteria=u2 > Threshold  SaturateOnIntegerOverflow=off  InputSameDT=off
  Switch1 : Switch  Criteria=u2 > Threshold  SaturateOnIntegerOverflow=off  InputSameDT=off
  "X " : Outport
  Z : Outport  Port=2
  wires:
  Swing Phase/1(X) -> Switch/1
  Swing Phase/2("Z ") -> Switch1/1
  Stance Phase/2("Z ") -> Switch1/3
  Stance Phase/1(X) -> Switch/3
  Divide1/1 -> Gain1/1
  Divide/1 -> Gain/1
  Duty Cycle/1 -> Subtract/2, Divide/2, Subsystem/2(Duty Cycle)
  Offset/1 -> Subsystem/3(Offset)
  Frequency/1 -> Divide1/1, Divide/1, Subsystem/1(Frequency)
  Subsystem/1(Swing Activation) -> Switch1/2, Switch/2, Swing Phase/Reset
  Subsystem/2(Stance Activation) -> Stance Phase/Reset
  Subtract/1 -> Divide1/2
  Constant2/1 -> Subtract/1
  Gain/1 -> Swing Phase/1(Frequency)
  Gain1/1 -> Stance Phase/1(Frequency)
  Switch1/1 -> Z/1
  Switch/1 -> "X "/1

== system HexapodLocomotion_Library/Swing-Stance Pattern Generation ==
  Cycle Frequency [Hz] : Inport
  Duty Cycle [%] : Inport  Port=2
  Initiate Swing : Inport  Port=3
  Determine Frequencies : Subsystem
  Swing-Stance Signal Generation : Subsystem
  X : Outport
  Z : Outport  Port=2
  wires:
  Swing-Stance Signal Generation/1(X) -> X/1
  Cycle Frequency [Hz]/1 -> Determine Frequencies/1(Cycle Frequency [Hz])
  Determine Frequencies/1(Swing Frequency [Hz]) -> Swing-Stance Signal Generation/1(Swing Frequency [Hz])
  Initiate Swing/1 -> Swing-Stance Signal Generation/3(Initiate Swing)
  Duty Cycle [%]/1 -> Determine Frequencies/2(Duty Cycle [%])
  Determine Frequencies/2(Stance Frequency [Hz]) -> Swing-Stance Signal Generation/2(Stance Frequency [Hz])
  Swing-Stance Signal Generation/2(Z) -> Z/1

== system HexapodLocomotion_Library/Ellipse Generation Freq. Coord. (Gen. 1)/If Action Subsystem ==
  Action Port : ActionPort
  Constant : Constant
  Out1 : Outport
  wires:
  Constant/1 -> Out1/1

== system HexapodLocomotion_Library/Ellipse Generation Freq. Coord. (Gen. 1)/If Action Subsystem1 ==
  Action Port : ActionPort
  Constant : Constant  Value=0
  Out1 : Outport
  wires:
  Constant/1 -> Out1/1

== system HexapodLocomotion_Library/Ellipse Generation Verschoben(Gen. 1)/If Action Subsystem ==
  Action Port : ActionPort
  Constant : Constant  Value=0
  Out1 : Outport
  wires:
  Constant/1 -> Out1/1

== system HexapodLocomotion_Library/Ellipse Generation Verschoben(Gen. 1)/If Action Subsystem1 ==
  Action Port : ActionPort
  Constant : Constant
  Out1 : Outport
  wires:
  Constant/1 -> Out1/1

== system HexapodLocomotion_Library/Ellipse Generation(Gen. 1)/If Action Subsystem ==
  Action Port : ActionPort
  Constant : Constant  Value=0
  Out1 : Outport
  wires:
  Constant/1 -> Out1/1

== system HexapodLocomotion_Library/Ellipse Generation(Gen. 1)/If Action Subsystem1 ==
  Action Port : ActionPort
  Constant : Constant
  Out1 : Outport
  wires:
  Constant/1 -> Out1/1
